simulink model "Aldovino_JYB_Simulink_No7"  (R2023b)
settings: Solver=VariableStepAuto  StartTime=0.0  StopTime=20.0  RelTol=1e-3
values from neighbouring files (symbols this model uses):
  G_den = [a b c]    [AGBAY_KZM_NO_1.m]    (also in AGBAY_KZM_NO_8.m = [f g h i j k]; ALDOVINO_JYB_NO_2.m = [M B k]; ALDOVINO_JYB_NO_7.m = [F G H I J K])
  G_num = [d]    [AGBAY_KZM_NO_1.m]    (also in AGBAY_KZM_NO_8.m = [a b c d e]; ALDOVINO_JYB_NO_2.m = [1]; ALDOVINO_JYB_NO_7.m = [A B C D E])
settings Model: Creator=User  LastModifiedBy=User

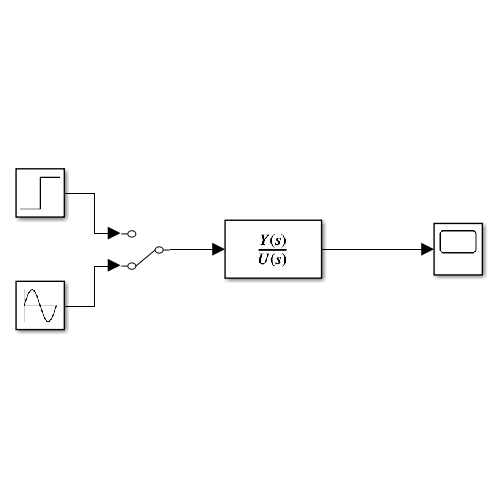
[thumbnail: Simulink's stored preview of the top-level diagram]
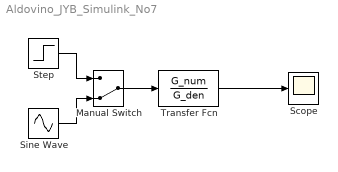
== system Aldovino_JYB_Simulink_No7 ==
  Manual Switch : ManualSwitch  CurrentSetting=0
  Scope : Scope
  Sine Wave : Sin  SampleTime=0
  Step : Step  Time=0  After=0  SampleTime=0
  Transfer Fcn : TransferFcn  Numerator=G_num  Denominator=G_den
  wires:
  Step/1 -> Manual Switch/1
  Transfer Fcn/1 -> Scope/1
  Manual Switch/1 -> Transfer Fcn/1
  Sine Wave/1 -> Manual Switch/2
